simulink model "Code2_simulink"  (R2016b)
settings: Solver=VariableStepAuto  StartTime=0.0  StopTime=10.0  RelTol=1e-3
settings Model: Creator=branden  LastModifiedBy=branden

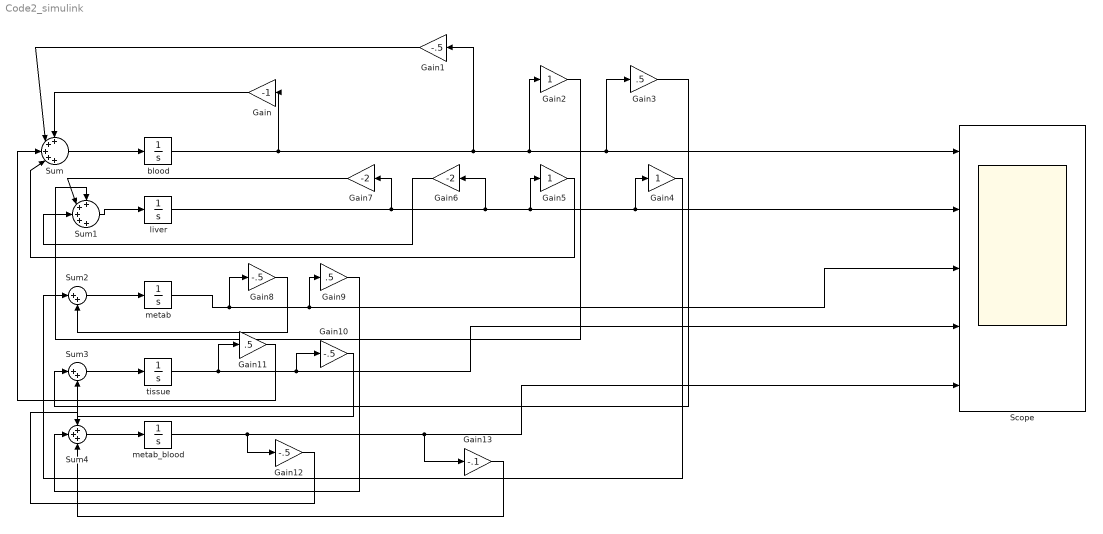
== system Code2_simulink ==
  Gain : Gain  Gain=-1
  Gain{1,8,10,12} (4 alike) : Gain  Gain=-.5
  Gain11 : Gain  Gain=.5
  Gain13 : Gain  Gain=-.1
  Gain2 : Gain
  Gain3 : Gain  Gain=.5
  Gain4 : Gain
  Gain5 : Gain
  Gain6 : Gain  Gain=-2
  Gain7 : Gain  Gain=-2
  Gain9 : Gain  Gain=.5
  Scope : Scope  NumInputPorts=5
  Sum : Sum  Inputs=+++++
  Sum1 : Sum  Inputs=+++++
  Sum2 : Sum  Inputs=|++
  Sum3 : Sum  Inputs=|++
  Sum4 : Sum  Inputs=+++
  blood : Integrator  InitialCondition=1000
  liver : Integrator
  "metab " : Integrator
  "metab_blood " : Integrator
  tissue : Integrator
  wires:
  blood/1 -> Gain/1, Gain1/1, Gain2/1, Gain3/1, Scope/1
  liver/1 -> Gain7/1, Gain6/1, Gain5/1, Gain4/1, Scope/2
  Gain/1 -> Sum/1
  Gain1/1 -> Sum/2
  Sum/1 -> blood/1
  Sum1/1 -> liver/1
  Sum2/1 -> "metab "/1
  Sum3/1 -> tissue/1
  Sum4/1 -> "metab_blood "/1
  Gain2/1 -> Sum1/1
  Gain3/1 -> Sum3/1
  Gain7/1 -> Sum1/2
  Gain6/1 -> Sum1/3
  Gain5/1 -> Sum/4
  Gain4/1 -> Sum2/1
  "metab "/1 -> Gain8/1, Gain9/1, Scope/3
  Gain8/1 -> Sum2/2
  Gain9/1 -> Sum4/2
  tissue/1 -> Gain11/1, Gain10/1, Scope/4
  Gain11/1 -> Sum/3
  Gain10/1 -> Sum3/2
  "metab_blood "/1 -> Gain12/1, Gain13/1, Scope/5
  Gain12/1 -> Sum4/1
  Gain13/1 -> Sum4/3
